simulink model "PCM_Simu"  (R2022a)
settings: Solver=VariableStepAuto  StartTime=0.0  StopTime=20  RelTol=1e-3
libraries: dspquant2 x2, dsparch4 x1, dspsigops x1
settings Model: Creator=HP  LastModifiedBy=HP

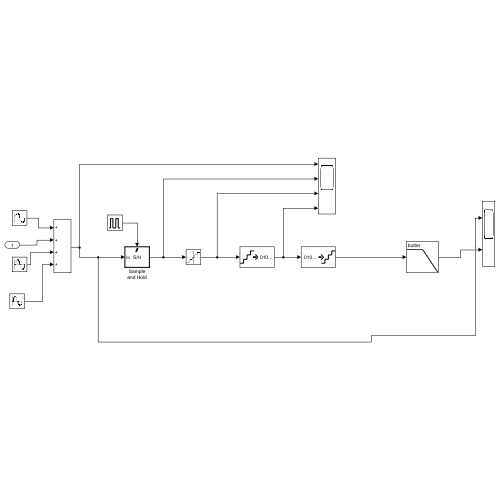
[thumbnail: Simulink's stored preview of the top-level diagram]
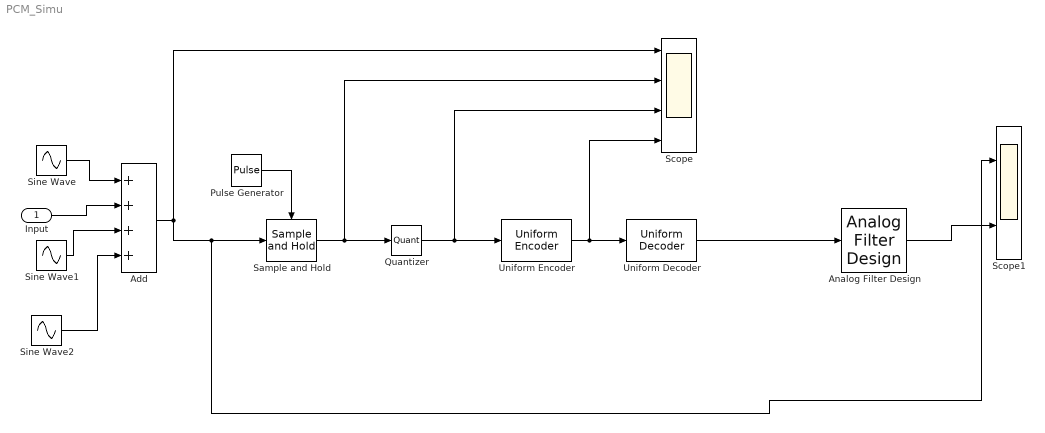
== system PCM_Simu ==
  Input : Inport
  Add : Sum  Inputs=++++
  Analog Filter Design : dsparch4/Analog Filter Design  method=Butterworth  filttype=Lowpass  N=8  Wlo=6  Whi=80  Rp=2  Rs=40
  Pulse Generator : DiscretePulseGenerator  PulseType=Time based  Period=0.1  PulseWidth=50
  Quantizer : Quantizer
  Sample and Hold : dspsigops/Sample and Hold  trig=Rising edge  initCond=0  latchinput=off
  Scope : Scope  NumInputPorts=4
  Scope1 : Scope  NumInputPorts=2
  Sine Wave : Sin  Frequency=6  SampleTime=1/10000
  Sine Wave1 : Sin  Amplitude=2.5  Frequency=4  Phase=pi*0.5  SampleTime=1/10000
  Sine Wave2 : Sin  Amplitude=sqrt(3)  Frequency=3  SampleTime=1/10000
  Uniform Decoder : dspquant2/Uniform Decoder  peak=5  bits=4  overflowMode=Saturate  otype=Double
      settings: SourceProductBaseCode=DS
  Uniform Encoder : dspquant2/Uniform Encoder  peak=5  bits=4  otype=Unsigned integer
  wires:
  Pulse Generator/1 -> Sample and Hold/Trigger
  Sample and Hold/1 -> Quantizer/1, Scope/2
  Quantizer/1 -> Uniform Encoder/1, Scope/3
  Sine Wave/1 -> Add/1
  Sine Wave1/1 -> Add/3
  Input/1 -> Add/2
  Sine Wave2/1 -> Add/4
  Uniform Encoder/1 -> Uniform Decoder/1, Scope/4
  Uniform Decoder/1 -> Analog Filter Design/1
  Analog Filter Design/1 -> Scope1/2
  Add/1 -> Scope/1, Scope1/1, Sample and Hold/1
